simulink model "ship_system"  (R2018b)
settings: Solver=VariableStepAuto  StartTime=0.0  StopTime=10.0  RelTol=1e-3
libraries: fl_lib x11, elec_lib x4, pe_lib x4
settings Model: Creator=hood000j  LastModifiedBy=hood000j

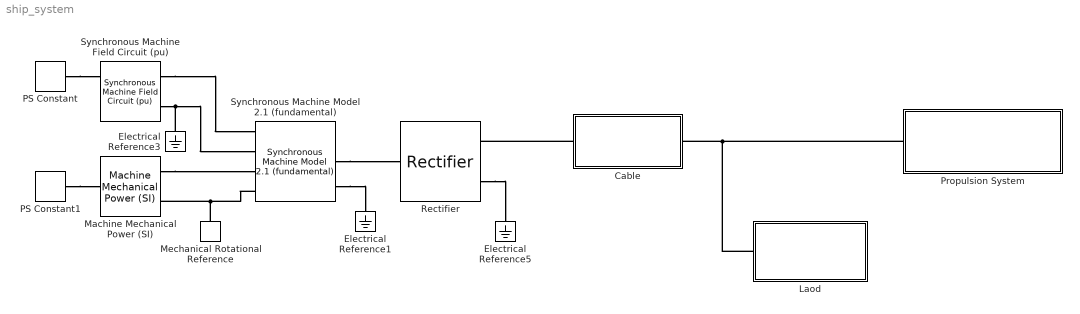
== system ship_system ==
  Cable : Subsystem
  Electrical Reference1 : fl_lib/Electrical/Electrical Elements/Electrical Reference
  Electrical Reference3 : fl_lib/Electrical/Electrical Elements/Electrical Reference
  Electrical Reference5 : fl_lib/Electrical/Electrical Elements/Electrical Reference
  Laod : Subsystem
  Machine Mechanical Power (SI) : pe_lib/Machines/Machine Mechanical Power (SI)  power_sign=-1  SRated=50e3 V*A  FRated=60 Hz  nPolePairs=1  torque_factor=2  inertia_option=2  J=27548 kg*m^2  H=10 s*W/V/A  damper_option=2  D=39.0509 N*m/(rad/s)  pu_D=0.01  initialization_option=2  fMechanical0=60 Hz  fElectrical0=60 Hz
      settings: SourceProductName=Simscape Power Systems  SourceProductBaseCode=PS
  Mechanical Rotational Reference : fl_lib/Mechanical/Rotational Elements/Mechanical Rotational Reference
  PS Constant : fl_lib/Physical Signals/Sources/PS Constant  constant=1
  PS Constant1 : fl_lib/Physical Signals/Sources/PS Constant  constant=50e3
  Propulsion System : Subsystem
  Rectifier : pe_lib/Semiconductors/Rectifier  model_dynamics=0  Vf=0.8 V  Ron=0.001 Ohm  Goff=1e-5 1/Ohm  C=50 nF  iRM=-235 A  iF=300 A  idot=-50 A/us  trr_param=1  trr_factor=3  trr=15 us  Qrr=1500 s*uA
      settings: SourceProductName=Simscape Power Systems  SourceProductBaseCode=PS
  Synchronous Machine Field Circuit (pu) : pe_lib/Machines/Synchronous Machine Field Circuit (pu)  SRated=50e6 V*A  FRated=60 Hz  fieldCircuitParameterization_option=2  baseEfd=92.95 V  baseIfd=500 A  parameterization_option=1  Ladu=1.66  Rfd=0.0006  Xl=0.15  Xd=1.81  Xdd=0.3  Xddd=0.23  d_option=1  Td0d=8 s  Tdd=1.3260 s  Td0dd=0.03 s  Tddd=0.0230 s
      settings: SourceProductName=Simscape Power Systems  SourceProductBaseCode=PS
  Synchronous Machine Model 2.1 (fundamental) : pe_lib/Machines/Synchronous Machine (Simplified)/Synchronous Machine Model 2.1 (fundamental)  SRated=50e6 V*A  VRated=4160 V  FRated=60 Hz  nPolePairs=1  fieldCircuitParameterization_option=2  baseEfd=92.95 V  baseIfd=500 A  Ladu=1.66  Laqu=1.61  Ll=0.15  Ra=0.003  Lfd=0.165  Rfd=0.0006  L1d=0.1713  R1d=0.0284  L1q=0.1066  R1q=0.0650  axes_param=pe.enum.rotorangle.daxis  initialization_option=2  angular_position0=0 deg  eddd0=0  eqd0=0  eqdd0=0  Vmag0=4160 V  Vang0=0 deg  Pt0=50e6 V*A  Qt0=0 V*A  connection_option=pe.Connection.wye  rotor_offset=-pi / 2 rad  num_q_dampers=1
      settings: SourceProductName=Simscape Power Systems  SourceProductBaseCode=PS
  connections:
  Synchronous Machine Model 2.1 (fundamental)/RConn3 -- Electrical Reference1/LConn1
  Machine Mechanical Power (SI)/RConn1 -- Synchronous Machine Model 2.1 (fundamental)/LConn3
  Synchronous Machine Model 2.1 (fundamental)/LConn4 -- Mechanical Rotational Reference/LConn1 -- Machine Mechanical Power (SI)/RConn2
  Synchronous Machine Field Circuit (pu)/RConn1 -- Synchronous Machine Model 2.1 (fundamental)/LConn1
  Synchronous Machine Field Circuit (pu)/RConn2 -- Synchronous Machine Model 2.1 (fundamental)/LConn2 -- Electrical Reference3/LConn1
  Synchronous Machine Model 2.1 (fundamental)/RConn2 -- Rectifier/LConn1
  Rectifier/RConn2 -- Electrical Reference5/LConn1
  PS Constant1/RConn1 -- Machine Mechanical Power (SI)/LConn1
  PS Constant/RConn1 -- Synchronous Machine Field Circuit (pu)/LConn1
  Laod/LConn1 -- Propulsion System/LConn1 -- Cable/RConn1
  Cable/LConn1 -- Rectifier/RConn1

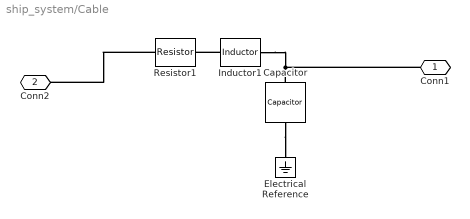
== system ship_system/Cable ==
  Capacitor : fl_lib/Electrical/Electrical Elements/Capacitor  c=1e-3 F  r=1e-6 Ohm  g=0 1/Ohm  i_specify=off  i_priority=None  i=0 A  i_nominal_specify=off  i_nominal_unit=A  i_nominal_value=1  v_specify=off  v_priority=None  v=0 V  v_nominal_specify=off  v_nominal_unit=V  v_nominal_value=1  vc_specify=off  vc_priority=High  vc=0 V  vc_nominal_specify=off  vc_nominal_unit=V  vc_nominal_value=1
  Electrical Reference : fl_lib/Electrical/Electrical Elements/Electrical Reference
  Inductor1 : fl_lib/Electrical/Electrical Elements/Inductor  l=1e-3 H  r=0 Ohm  g=1e-9 1/Ohm  i_specify=off  i_priority=None  i=0 A  i_nominal_specify=off  i_nominal_unit=A  i_nominal_value=1  v_specify=off  v_priority=None  v=0 V  v_nominal_specify=off  v_nominal_unit=V  v_nominal_value=1  i_L_specify=off  i_L_priority=High  i_L=0 A  i_L_nominal_specify=off  i_L_nominal_unit=A  i_L_nominal_value=1
  Resistor1 : fl_lib/Electrical/Electrical Elements/Resistor  R=0.01 Ohm  i_specify=off  i_priority=None  i=0 A  i_nominal_specify=off  i_nominal_unit=A  i_nominal_value=1  v_specify=off  v_priority=None  v=0 V  v_nominal_specify=off  v_nominal_unit=V  v_nominal_value=1
  Conn1 : PMIOPort  Side=Right
  Conn2 : PMIOPort  Port=2  Side=Left
  connections:
  Inductor1/LConn1 -- Resistor1/RConn1
  Inductor1/RConn1 -- Conn1/RConn1 -- Capacitor/LConn1
  Resistor1/LConn1 -- Conn2/RConn1
  Capacitor/RConn1 -- Electrical Reference/LConn1

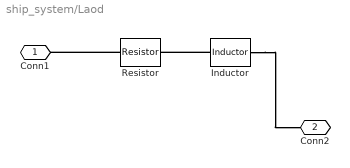
== system ship_system/Laod ==
  Inductor : elec_lib/Passive Devices/Inductor  l=1e-6 H  L_tol=20  enable_L_tol=0  tol_distribution=1  nSigma=4  r=0 Ohm  g=1e-9 1/Ohm  enable_operating_limits=0  operating_limit_action=2  max_working_current=1 A  power_rating=1 W  enable_faults=0  fault_action=1  lambdaPercent=50  k_faulted=0.9999  turnsShort=0  openCct=0  groundShort=0  groundShortG=0 1/Ohm  tau_fault=1e-3 s  enable_temporal_fault=0  t_fault=1 s  enable_behavioral_fault=0  max_permissible_voltage=100 V  n_fail_on_voltage=1  max_permissible_current=1 A  t_fail_on_current=1 s  i_L_specify=off  i_L_priority=High  i_L=0 A  i_L_nominal_specify=off  i_L_nominal_unit=A  i_L_nominal_value=1
      settings: SourceProductName=Simscape Electronics  SourceProductBaseCode=SN
  Resistor : elec_lib/Passive Devices/Resistor  R=1 Ohm  R_tol=5  enable_R_tol=0  tol_distribution=1  nSigma=4  enable_operating_limits=0  operating_limit_action=2  max_working_voltage=100 V  power_rating=1 W  enable_faults=0  fault_action=1  R_faulted=inf Ohm  enable_temporal_fault=0  t_fault=1 s  enable_behavioral_fault=0  max_permissible_current=1 A  t_fail_on_current=1 s  noise_mode=0  sample_time=1e-3 s  repeatability=1  auto_seed=3890346746  user_seed=0  Tdevice=25 degC  alpha=3.93e-3 1/K  Tmeas=25 degC  thermal_mass=100 J/K  power_derating_T1=70 degC  power_derating_T2=155 degC  operating_temperature_range_vec=[-50, 150] degC  temperature_specify=off  temperature_priority=High  temperature=298.15 K  temperature_nominal_specify=off  temperature_nominal_unit=K  temperature_nominal_value=1
  Conn1 : PMIOPort  Side=Left
  Conn2 : PMIOPort  Port=2  Side=Right
  connections:
  Resistor/LConn1 -- Conn1/RConn1
  Inductor/LConn1 -- Resistor/RConn1
  Inductor/RConn1 -- Conn2/RConn1

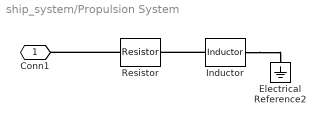
== system ship_system/Propulsion System ==
  Electrical Reference2 : fl_lib/Electrical/Electrical Elements/Electrical Reference
  Inductor : elec_lib/Passive Devices/Inductor  l=1e-6 H  L_tol=20  enable_L_tol=0  tol_distribution=1  nSigma=4  r=0 Ohm  g=1e-9 1/Ohm  enable_operating_limits=0  operating_limit_action=2  max_working_current=1 A  power_rating=1 W  enable_faults=0  fault_action=1  lambdaPercent=50  k_faulted=0.9999  turnsShort=0  openCct=0  groundShort=0  groundShortG=0 1/Ohm  tau_fault=1e-3 s  enable_temporal_fault=0  t_fault=1 s  enable_behavioral_fault=0  max_permissible_voltage=100 V  n_fail_on_voltage=1  max_permissible_current=1 A  t_fail_on_current=1 s  i_L_specify=off  i_L_priority=High  i_L=0 A  i_L_nominal_specify=off  i_L_nominal_unit=A  i_L_nominal_value=1
      settings: SourceProductName=Simscape Electronics  SourceProductBaseCode=SN
  Resistor : elec_lib/Passive Devices/Resistor  R=1 Ohm  R_tol=5  enable_R_tol=0  tol_distribution=1  nSigma=4  enable_operating_limits=0  operating_limit_action=2  max_working_voltage=100 V  power_rating=1 W  enable_faults=0  fault_action=1  R_faulted=inf Ohm  enable_temporal_fault=0  t_fault=1 s  enable_behavioral_fault=0  max_permissible_current=1 A  t_fail_on_current=1 s  noise_mode=0  sample_time=1e-3 s  repeatability=1  auto_seed=3005995426  user_seed=0  Tdevice=25 degC  alpha=3.93e-3 1/K  Tmeas=25 degC  thermal_mass=100 J/K  power_derating_T1=70 degC  power_derating_T2=155 degC  operating_temperature_range_vec=[-50, 150] degC  temperature_specify=off  temperature_priority=High  temperature=298.15 K  temperature_nominal_specify=off  temperature_nominal_unit=K  temperature_nominal_value=1
  Conn1 : PMIOPort  Side=Left
  connections:
  Resistor/LConn1 -- Conn1/RConn1
  Inductor/LConn1 -- Resistor/RConn1
  Inductor/RConn1 -- Electrical Reference2/LConn1
